simulink model "Q2_SIM"  (R2021b)
settings: Solver=VariableStepAuto  StartTime=0.0  StopTime=1  RelTol=1e-3
undefined symbols (not defined in the file): Gc, gp
settings Model: Creator=Lenovo  LastModifiedBy=Lenovo

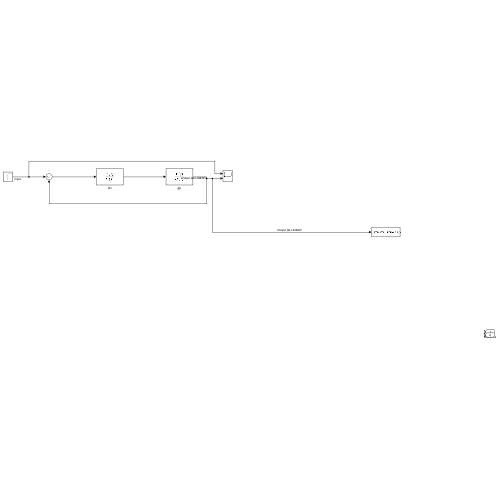
[thumbnail: Simulink's stored preview of the top-level diagram]
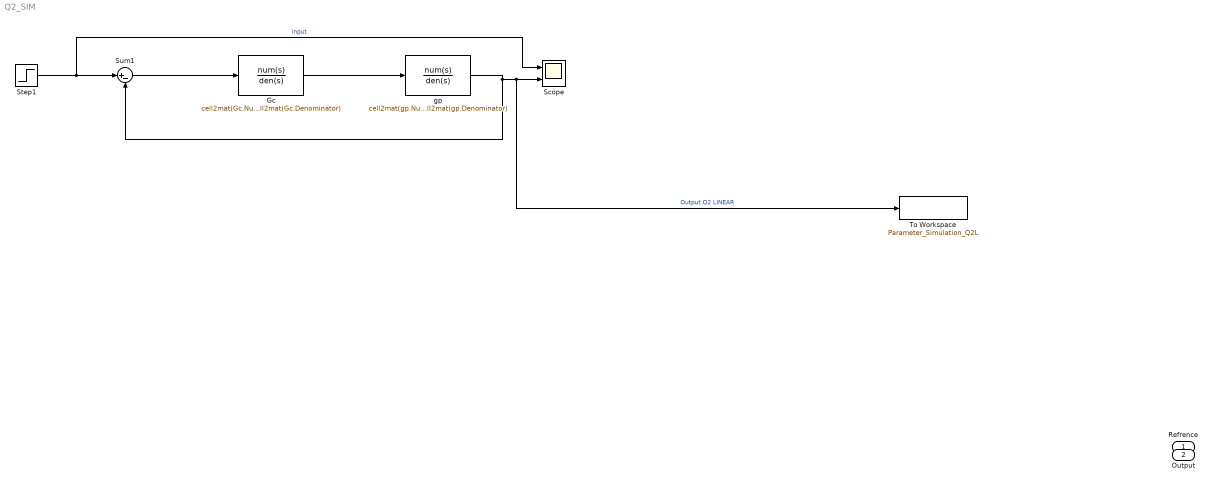
== system Q2_SIM ==
  Gc : TransferFcn  Numerator=cell2mat(Gc.Numerator)  Denominator=cell2mat(Gc.Denominator)
  Scope : Scope  NumInputPorts=2
  Step1 : Step  Time=0  After=0.0001  SampleTime=0
  Sum1 : Sum  Inputs=|+-
  To Workspace : ToWorkspace  VariableName=Parameter_Simulation_Q2L  SaveFormat=Timeseries  SampleTime=-1
  gp : TransferFcn  Numerator=cell2mat(gp.Numerator)  Denominator=cell2mat(gp.Denominator)
  Refrence : Outport
  Output : Outport  Port=2
  wires:
  Sum1/1 -> Gc/1
  Step1/1 -> Scope/1, Sum1/1  "input"
  Gc/1 -> gp/1
  gp/1 -> Sum1/2, To Workspace/1, Scope/2  "Output Q2 LINEAR"
